simulink model "Single1"  (R2016a)
settings: Solver=FixedStepDiscrete  StartTime=0.0  StopTime=400e-9  FixedStep=SampleTime  RelTol=1e-3
values from neighbouring files (symbols this model uses):
  Rd = (3.6/4) * (0.95*0.82*(1 - (-0.0128*(Temp - 25))) * 18.2 / 295) + 1e-4    (= 0.11256119322)    [DPTThermalGaNModel.m]    (also in Thermal_CurrentVoltageGraph.m = (3.6/4) * (0.95*0.82*(1 - (-0.0128*(Temp(TempIndex) - 25))) )
  Rs = 3.6 * 0.238 * 0.82 * (1 - (-0.0128*(Temp - 25))) / 295 + 1e-4    (= 0.00629219525424)    [DPTThermalGaNModel.m]    (also in Thermal_CurrentVoltageGraph.m = 3.6 * 0.238 * 0.82 * (1 - (-0.0128*(Temp(TempIndex) - 25))) )
  Rss = 1e-3    (= 0.001)    [DPTThermalGaNModel.m]
  VpulseMax = 6    [DPTThermalGaNModel.m]
undefined symbols (not defined in the file or in its folder): Rgin
libraries: elec_lib x16, nesl_utility x15, fl_lib x14
settings Model: Creator=ugurm  LastModifiedBy=Furkan
settings OptimizationCC: EfficientMapNaN2IntZero=off
settings HardwareCC: TargetBitPerPointer=64  TargetLongLongMode=on  TargetIntDivRoundTo=Zero  TargetEndianess=LittleEndian  TargetWordSize=64  TargetHWDeviceType=MATLAB Host  ProdEqTarget=off
settings CodeAppCC: MaxIdLength=128
settings GRTTargetCC: GeneratePreprocessorConditionals=Use local settings  CombineOutputUpdateFcns=off  GRTInterface=on

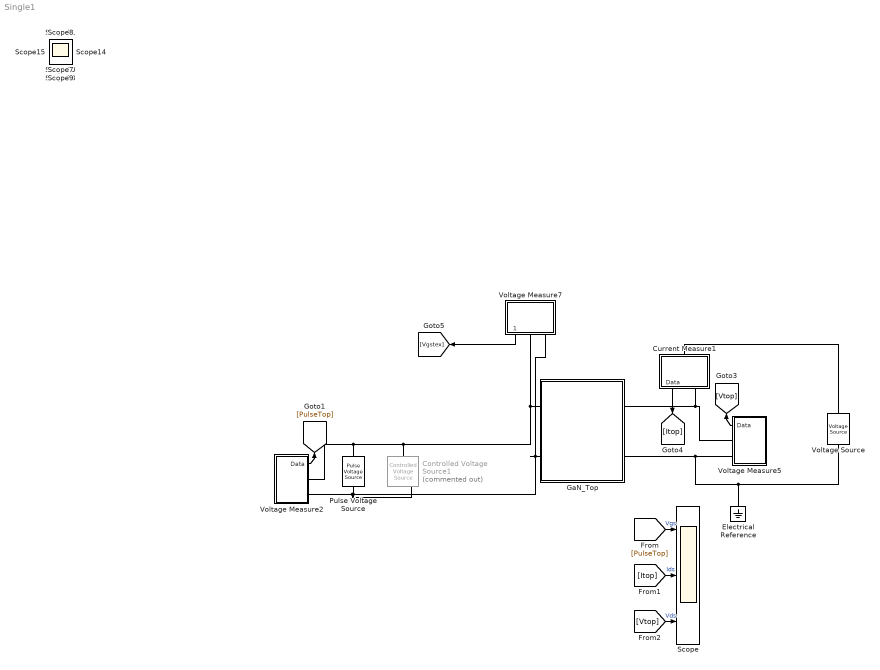
== system Single1 ==
  Controlled Voltage Source1 : fl_lib/Electrical/Electrical Sources/Controlled Voltage Source  Commented=on
  Current Measure1 : Subsystem
  Electrical Reference : fl_lib/Electrical/Electrical Elements/Electrical Reference
  GaN_Top : Subsystem
  Pulse Voltage Source : elec_lib/Additional Components/SPICE-Compatible Components/Sources/Pulse Voltage Source  V1=-3 V  V2=6 V  TD=50e-9 s  TR=1e-10 s  TF=1e-10 s  PW=150e-9 s  PER=500e-9 s
  Scope : Scope  NumInputPorts=3
  Voltage Measure2 : Subsystem
  Voltage Measure5 : Subsystem
  Voltage Measure7 : Subsystem
  Voltage Source : elec_lib/Sources/Voltage Source  dc_voltage=2 V  ac_voltage=0 V  ac_shift=0 deg  ac_frequency=60 Hz  noise_mode=0  PSD=0 V^2/Hz  sample_time=0.001 s  repeatability=1  auto_seed=3499211588  user_seed=0
  Scope{7..11,13..15} (8 alike) : Scope
  wires:
  Voltage Measure2/1(Data) -> [PulseTop]
  Voltage Measure5/1(Data) -> [Vtop]
  Current Measure1/1(Data) -> [Itop]
  Voltage Measure7/1(Data) -> [Vgstex]
  [PulseTop] -> Scope/1  "Vgs"
  [Itop] -> Scope/2  "Ids"
  [Vtop] -> Scope/3  "Vds"
  connections:
  GaN_Top/LConn1 -- Voltage Measure2/RConn1 -- Pulse Voltage Source/LConn1 -- Controlled Voltage Source1/LConn1 -- Voltage Measure7/RConn1
  GaN_Top/RConn1 -- Current Measure1/RConn1 -- Voltage Measure5/RConn1
  Pulse Voltage Source/RConn1 -- Controlled Voltage Source1/RConn2 -- Voltage Measure2/RConn2 -- GaN_Top/LConn2 -- Voltage Measure7/RConn2
  GaN_Top/RConn2 -- Electrical Reference/LConn1 -- Voltage Source/RConn1 -- Voltage Measure5/RConn2
  Voltage Source/LConn1 -- Current Measure1/LConn1

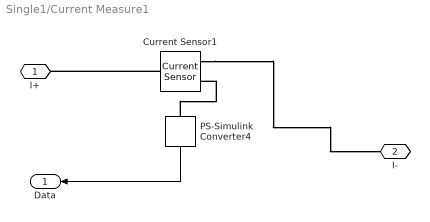
== system Single1/Current Measure1 ==
  Current Sensor1 : fl_lib/Electrical/Electrical Sensors/Current Sensor
  PS-Simulink Converter4 : nesl_utility/PS-Simulink Converter  PhysicalDomain=network_engine_domain  SubClassName=ps_output  LeftPortType=input  RightPortType=output  PseudoPeriodic=off  Frequencies=[]  Unit=1  AffineConversion=off
  I+ : PMIOPort  Port=1  Side=Left
  I- : PMIOPort  Port=2  Side=Right
  Data : Outport
  wires:
  PS-Simulink Converter4/1 -> Data/1
  connections:
  Current Sensor1/RConn2 -- I-/RConn1
  PS-Simulink Converter4/LConn1 -- Current Sensor1/RConn1
  Current Sensor1/LConn1 -- I+/RConn1

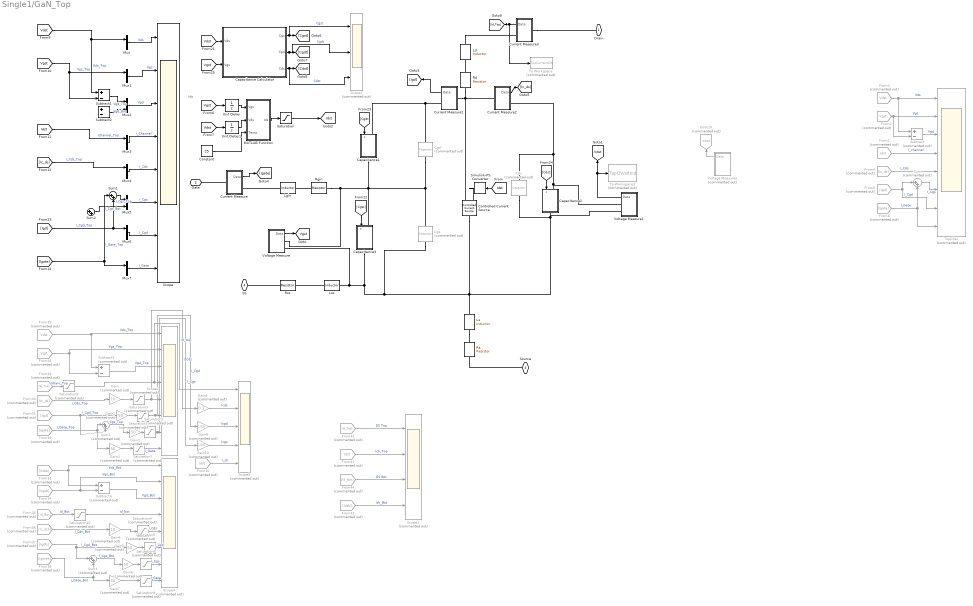
== system Single1/GaN_Top ==
  note: Ids
  Capacitance Calculator : Subsystem
  Capacitance1 : Subsystem
  Capacitance2 : Subsystem
  Capacitance3 : Subsystem
  Cds : elec_lib/Passive Devices/Capacitor  Commented=on  enable_table=0  c=Cds F  Cvec=[ 1e-5 1e-6 ] F  Vvec=[ 0 10 ] V  CV_table_symmetry=1  C_tol=5  enable_C_tol=0  tol_distribution=1  nSigma=4  r=1e-6 Ohm  g=0 1/Ohm  initV=VoltDSTop V  enable_operating_limits=0  operating_limit_action=2  max_working_voltage_range=[ -25 25 ] V  power_rating=1 W  enable_faults=0  fault_action=1  Cscale_faulted=100  R_faulted=0.001 Ohm  G_faulted=0 1/Ohm  tau_fault=0.001 s  enable_temporal_fault=0  t_fault=1 s  enable_behavioral_fault=0  max_permissible_voltage_range=[ -100 100 ] V  t_fail_on_voltage=1 s
  Cgd : elec_lib/Passive Devices/Capacitor  Commented=on  enable_table=0  c=Cgd F  Cvec=[ 1e-5 1e-6 ] F  Vvec=[ 0 10 ] V  CV_table_symmetry=1  C_tol=5  enable_C_tol=0  tol_distribution=1  nSigma=4  r=1e-6 Ohm  g=0 1/Ohm  initV=-VpulseMax V  enable_operating_limits=0  operating_limit_action=2  max_working_voltage_range=[ -25 25 ] V  power_rating=1 W  enable_faults=0  fault_action=1  Cscale_faulted=100  R_faulted=0.001 Ohm  G_faulted=0 1/Ohm  tau_fault=0.001 s  enable_temporal_fault=0  t_fault=1 s  enable_behavioral_fault=0  max_permissible_voltage_range=[ -100 100 ] V  t_fail_on_voltage=1 s
  Cgs : elec_lib/Passive Devices/Capacitor  Commented=on  enable_table=0  c=Cgs F  Cvec=[ 1e-5 1e-6 ] F  Vvec=[ 0 10 ] V  CV_table_symmetry=1  C_tol=5  enable_C_tol=0  tol_distribution=1  nSigma=4  r=1e-6 Ohm  g=0 1/Ohm  initV=VpulseMin V  enable_operating_limits=0  operating_limit_action=2  max_working_voltage_range=[ -25 25 ] V  power_rating=1 W  enable_faults=0  fault_action=1  Cscale_faulted=100  R_faulted=0.001 Ohm  G_faulted=0 1/Ohm  tau_fault=0.001 s  enable_temporal_fault=0  t_fault=1 s  enable_behavioral_fault=0  max_permissible_voltage_range=[ -100 100 ] V  t_fail_on_voltage=1 s
  Constant : Constant  Value=25
  Controlled Current Source : fl_lib/Electrical/Electrical Sources/Controlled Current Source
  Current Measure : Subsystem
  Current Measure1 : Subsystem
  Current Measure2 : Subsystem
  Current Measure3 : Subsystem
  From1 : From  Commented=on  GotoTag=Idst  TagVisibility=global
  From2 : From  Commented=on  GotoTag=Vgst  TagVisibility=global
  From28 : From  Commented=on  GotoTag=Vgst  TagVisibility=global
  From29 : From  Commented=on  GotoTag=Id_Top
  From3 : From  Commented=on  GotoTag=Vdst  TagVisibility=global
  From30 : From  Commented=on  GotoTag=Ic_ds
  From31 : From  Commented=on  GotoTag=Igd
  From32 : From  Commented=on  GotoTag=Igate
  From33 : From  Commented=on  GotoTag=Vdsb  TagVisibility=global
  From34 : From  Commented=on  GotoTag=Vgsb  TagVisibility=global
  From35 : From  Commented=on  GotoTag=Id_Bot  TagVisibility=global
  From36 : From  Commented=on  GotoTag=Ic_dsb  TagVisibility=global
  From37 : From  Commented=on  GotoTag=Igdb  TagVisibility=global
  From38 : From  Commented=on  GotoTag=Igateb  TagVisibility=global
  From39 : From  Commented=on  GotoTag=Vdst  TagVisibility=global
  From4 : From  Commented=on  GotoTag=Ic_ds
  From40 : From  Commented=on  GotoTag=Idst  TagVisibility=global
  From41 : From  Commented=on  GotoTag=Idst  TagVisibility=global
  From42 : From  Commented=on  GotoTag=Idsb  TagVisibility=global
  From43 : From  Commented=on  GotoTag=Id_Top
  From44 : From  Commented=on  GotoTag=Id_Bot  TagVisibility=global
  From5 : From  Commented=on  GotoTag=Igd
  From8 : From  Commented=on  GotoTag=Igate
  Gain : Gain  Commented=on  Gain=10
  Gain{1..3,5..7} (6 alike) : Gain  Commented=on  Gain=50
  Gain10 : Gain  Commented=on  Gain=1/50
  Gain4 : Gain  Commented=on  Gain=10
  Gain8 : Gain  Commented=on  Gain=0.1
  Gain9 : Gain  Commented=on  Gain=1/50
  Goto10 : Goto  Commented=on  GotoTag=Vdsit  TagVisibility=global
  Ld : elec_lib/Passive Devices/Inductor  l=Ld H  L_tol=20  enable_L_tol=0  tol_distribution=1  nSigma=4  r=0 Ohm  g=1e-9 1/Ohm  initI=CurrDSTop A  enable_operating_limits=0  operating_limit_action=2  max_working_current=1 A  power_rating=1 W  enable_faults=0  fault_action=1  lambdaPercent=50  k_faulted=0.9999 Ohm  turnsShort=0  openCct=0  groundShort=0  groundShortG=0 1/Ohm  tau_fault=0.001 s  enable_temporal_fault=0  t_fault=1 s  enable_behavioral_fault=0  max_permissible_voltage=100 V  n_fail_on_voltage=1  max_permissible_current=1 A  t_fail_on_current=1 s
  "Lgin " : elec_lib/Passive Devices/Inductor  l=Lgin H  L_tol=20  enable_L_tol=0  tol_distribution=1  nSigma=4  r=0 Ohm  g=1e-9 1/Ohm  initI=0 A  enable_operating_limits=0  operating_limit_action=2  max_working_current=1 A  power_rating=1 W  enable_faults=0  fault_action=1  lambdaPercent=50  k_faulted=0.9999 Ohm  turnsShort=0  openCct=0  groundShort=0  groundShortG=0 1/Ohm  tau_fault=0.001 s  enable_temporal_fault=0  t_fault=1 s  enable_behavioral_fault=0  max_permissible_voltage=100 V  n_fail_on_voltage=1  max_permissible_current=1 A  t_fail_on_current=1 s
  Ls : elec_lib/Passive Devices/Inductor  l=Ls H  L_tol=20  enable_L_tol=0  tol_distribution=1  nSigma=4  r=0 Ohm  g=1e-9 1/Ohm  initI=CurrDSTop A  enable_operating_limits=0  operating_limit_action=2  max_working_current=1 A  power_rating=1 W  enable_faults=0  fault_action=1  lambdaPercent=50  k_faulted=0.9999 Ohm  turnsShort=0  openCct=0  groundShort=0  groundShortG=0 1/Ohm  tau_fault=0.001 s  enable_temporal_fault=0  t_fault=1 s  enable_behavioral_fault=0  max_permissible_voltage=100 V  n_fail_on_voltage=1  max_permissible_current=1 A  t_fail_on_current=1 s
  Lss : elec_lib/Passive Devices/Inductor  l=Lss H  L_tol=20  enable_L_tol=0  tol_distribution=1  nSigma=4  r=0 Ohm  g=1e-9 1/Ohm  initI=0 A  enable_operating_limits=0  operating_limit_action=2  max_working_current=1 A  power_rating=1 W  enable_faults=0  fault_action=1  lambdaPercent=50  k_faulted=0.9999 Ohm  turnsShort=0  openCct=0  groundShort=0  groundShortG=0 1/Ohm  tau_fault=0.001 s  enable_temporal_fault=0  t_fault=1 s  enable_behavioral_fault=0  max_permissible_voltage=100 V  n_fail_on_voltage=1  max_permissible_current=1 A  t_fail_on_current=1 s
  MATLAB Function : MATLAB Function  TreatAsAtomicUnit=on
  Mux{,1..7} (8 alike) : Mux  Inputs=2
  Rd : elec_lib/Passive Devices/Resistor  R=Rd Ohm  R_tol=5  enable_R_tol=0  tol_distribution=1  nSigma=4  enable_operating_limits=0  operating_limit_action=2  max_working_voltage=100 V  power_rating=1 W  enable_faults=0  fault_action=1  R_faulted=Inf Ohm  enable_temporal_fault=0  t_fault=1 s  enable_behavioral_fault=0  max_permissible_current=1 A  t_fail_on_current=1 s  noise_mode=0  sample_time=0.001 s  repeatability=1  auto_seed=1426435484  user_seed=0  Tdevice=25 degC  alpha=0.00393 1/K  Tmeas=25 degC  thermal_mass=100 J/K  initial_temperature=25 degC  power_derating_T1=70 degC  power_derating_T2=155 degC  operating_temperature_range_vec=[ -50 150 ] degC
  "Rgin " : elec_lib/Passive Devices/Resistor  R=Rgin Ohm  R_tol=5  enable_R_tol=0  tol_distribution=1  nSigma=4  enable_operating_limits=0  operating_limit_action=2  max_working_voltage=100 V  power_rating=1 W  enable_faults=0  fault_action=1  R_faulted=Inf Ohm  enable_temporal_fault=0  t_fault=1 s  enable_behavioral_fault=0  max_permissible_current=1 A  t_fail_on_current=1 s  noise_mode=0  sample_time=0.001 s  repeatability=1  auto_seed=2715962282  user_seed=0  Tdevice=25 degC  alpha=0.00393 1/K  Tmeas=25 degC  thermal_mass=100 J/K  initial_temperature=25 degC  power_derating_T1=70 degC  power_derating_T2=155 degC  operating_temperature_range_vec=[ -50 150 ] degC
  Rs : elec_lib/Passive Devices/Resistor  R=Rs Ohm  R_tol=5  enable_R_tol=0  tol_distribution=1  nSigma=4  enable_operating_limits=0  operating_limit_action=2  max_working_voltage=100 V  power_rating=1 W  enable_faults=0  fault_action=1  R_faulted=Inf Ohm  enable_temporal_fault=0  t_fault=1 s  enable_behavioral_fault=0  max_permissible_current=1 A  t_fail_on_current=1 s  noise_mode=0  sample_time=0.001 s  repeatability=1  auto_seed=3428974147  user_seed=0  Tdevice=25 degC  alpha=0.00393 1/K  Tmeas=25 degC  thermal_mass=100 J/K  initial_temperature=25 degC  power_derating_T1=70 degC  power_derating_T2=155 degC  operating_temperature_range_vec=[ -50 150 ] degC
  Rss : elec_lib/Passive Devices/Resistor  R=Rss Ohm  R_tol=5  enable_R_tol=0  tol_distribution=1  nSigma=4  enable_operating_limits=0  operating_limit_action=2  max_working_voltage=100 V  power_rating=1 W  enable_faults=0  fault_action=1  R_faulted=Inf Ohm  enable_temporal_fault=0  t_fault=1 s  enable_behavioral_fault=0  max_permissible_current=1 A  t_fail_on_current=1 s  noise_mode=0  sample_time=0.001 s  repeatability=1  auto_seed=299565776  user_seed=0  Tdevice=25 degC  alpha=0.00393 1/K  Tmeas=25 degC  thermal_mass=100 J/K  initial_temperature=25 degC  power_derating_T1=70 degC  power_derating_T2=155 degC  operating_temperature_range_vec=[ -50 150 ] degC
  Saturation : Saturate  UpperLimit=200  LowerLimit=-200
  Saturation{1..2,5..10} (8 alike) : Saturate  Commented=on  UpperLimit=100  LowerLimit=-100
  Saturation3 : Saturate  Commented=on  UpperLimit=250  LowerLimit=-100
  Saturation4 : Saturate  Commented=on  UpperLimit=250  LowerLimit=-100
  Scope : Scope  NumInputPorts=8
  Scope1 : Scope  Commented=on  NumInputPorts=3
  Scope2 : Scope  Commented=on  NumInputPorts=8
  Scope3 : Scope  Commented=on  NumInputPorts=4
  Scope4 : Scope  Commented=on  NumInputPorts=8
  Scope5 : Scope  Commented=on  NumInputPorts=5
  Simulink-PS Converter : nesl_utility/Simulink-PS Converter  PhysicalDomain=network_engine_domain  SubClassName=ps_input  LeftPortType=input  RightPortType=output  PseudoPeriodic=off  Frequencies=[]  NoiseDistribution=none  NoiseParameters=[]  Unit=1  AffineConversion=off  InputFiltering=off  SimscapeFilterOrder=1  InputFilterTimeConstant=0.001  UdotUserProvided=1
  Subtract : Sum  Commented=on  Inputs=+-
  Subtract1 : Sum  Inputs=+-
  Subtract2 : Sum  Inputs=+-
  Subtract3 : Sum  Commented=on  Inputs=+-
  Subtract4 : Sum  Commented=on  Inputs=+-
  Sum : Sum  Commented=on  Inputs=|++
  Sum1 : Sum  Inputs=|++
  Sum2 : Sum  Inputs=|++
  Sum3 : Sum  Commented=on  Inputs=|++
  Sum4 : Sum  Commented=on  Inputs=|++
  To Workspace : ToWorkspace  Commented=on  VariableName=TopCurrentDS  SampleTime=-1
      settings: Save2DSignal=2-D array (concatenate along first dimension)
  To Workspace3 : ToWorkspace  Commented=on  VariableName=TopChVoltInd  SampleTime=-1
      settings: Save2DSignal=2-D array (concatenate along first dimension)
  TopChar : Scope  Commented=on  NumInputPorts=8
  Unit Delay : UnitDelay  SampleTime=-1
  Unit Delay1 : UnitDelay  SampleTime=-1
  Voltage Measure : Subsystem
  Voltage Measure1 : Subsystem
  Voltage Measure2 : Subsystem  Commented=on
  Drain : PMIOPort  Port=1  Side=Right
  Gate : PMIOPort  Port=2  Side=Left
  Source : PMIOPort  Port=3  Side=Right
  SS : PMIOPort  Port=4  Side=Left
  tag scope: Idst=global, Vdst=global, Vgst=global
  wires:
  [Vgst] -> Unit Delay/1
  MATLAB Function/1(Ids) -> Saturation/1
  Unit Delay/1 -> MATLAB Function/1(Vgs)
  [Idst] -> Simulink-PS Converter/1
  From2/1 -> Subtract/2, TopChar/2  "Vgs"
  From3/1 -> Subtract/1, TopChar/1  "Vds"
  From1/1 -> TopChar/4  "I_channel"
  Subtract/1 -> TopChar/3  "Vgd"
  Current Measure1/1(Data) -> [Igd]
  Current Measure2/1(Data) -> [Ic_ds]
  From5/1 -> TopChar/7, Sum/1  "I_Cgd"
  From8/1 -> TopChar/8, Sum/2  "I_Gate"
  From4/1 -> TopChar/5  "I_Cds"
  Sum/1 -> TopChar/6  "I_Cgs"
  Current Measure/1(Data) -> [Igate]
  Voltage Measure/1(Data) -> [Vgst]
  [Vdst] -> Mux/1, Subtract1/1  "Vds_Top"
  [Vgst] -> Mux1/1, Subtract1/2  "Vgs_Top"
  [Ic_ds] -> Mux4/1  "I_Cds_Top"
  [Igd] -> Mux6/1, Sum1/2  "I_Cgd_Top"
  [Igate] -> Mux7/1, Sum1/1  "I_Gate_Top"
  Sum1/1 -> Mux5/1  "I_Cgs_Top"
  ? -> Subtract2/1, Mux/2  "Vds_Bot"
  ? -> Mux1/2, Subtract2/2  "Vgs_Bot"
  ? -> Mux4/2  "I_Cds_Bot"
  ? -> Mux6/2, Sum2/1  "I_Cgd_Bot"
  ? -> Mux7/2, Sum2/2  "I_Gate_Bot"
  Sum2/1 -> Mux5/2  "I_Cgs_Bot"
  Subtract1/1 -> Mux2/1  "Vgd_Top"
  Subtract2/1 -> Mux2/2  "Vgd_Bot"
  [Idst] -> Mux3/1  "Ichannel_Top"
  ? -> Mux3/2  "Ichannel_Bot"
  Mux7/1 -> Scope/8  "I_Gate"
  Mux6/1 -> Scope/7  "I_Cgd"
  Mux5/1 -> Scope/6  "I_Cgs"
  Mux4/1 -> Scope/5  "I_Cds"
  Mux3/1 -> Scope/4  "I_Channel"
  Mux2/1 -> Scope/3  "Vgd"
  Mux1/1 -> Scope/2  "Vgs"
  Mux/1 -> Scope/1  "Vds"
  [Vdst] -> Capacitance Calculator/1(Vds)
  Capacitance Calculator/1(Cgs) -> Scope1/1, [Cgst]  "Cgst"
  Capacitance Calculator/2(Cgd) -> Scope1/2, [Cgdt]  "Cgdt"
  Capacitance Calculator/3(Cds) -> Scope1/3, [Cdst]  "Cdst"
  [Cgst] -> Capacitance3/1(c)
  [Cgdt] -> Capacitance1/1(c)
  [Cdst] -> Capacitance2/1(c)
  From39/1 -> Scope2/1, Subtract3/1  "Vds_Top"
  From28/1 -> Scope2/2, Subtract3/2  "Vgs_Top"
  From30/1 -> Gain/1  "I_Cds_Top"
  From31/1 -> Sum3/2, Gain1/1  "I_Cgd_Top"
  From32/1 -> Gain3/1, Sum3/1  "I_Gate_Top"
  From33/1 -> Scope4/1, Subtract4/1  "Vds_Bot"
  From34/1 -> Scope4/2, Subtract4/2  "Vgs_Bot"
  From36/1 -> Gain4/1  "I_Cds_Bot"
  From37/1 -> Sum4/1, Gain5/1  "I_Cgd_Bot"
  From38/1 -> Gain7/1, Sum4/2  "I_Gate_Bot"
  Subtract3/1 -> Scope2/3  "Vgd_Top"
  Subtract4/1 -> Scope4/3  "Vgd_Bot"
  From29/1 -> Saturation9/1  "Idrain_Top"
  From35/1 -> Saturation10/1  "Id_Bot"
  Sum4/1 -> Gain6/1  "I_Cgs_Bot"
  Gain/1 -> Saturation3/1
  Gain1/1 -> Saturation2/1
  Sum3/1 -> Gain2/1  "I_Cgs_Top"
  Gain3/1 -> Saturation7/1
  Gain4/1 -> Saturation4/1
  Gain6/1 -> Saturation6/1
  Gain7/1 -> Saturation8/1
  Gain2/1 -> Saturation1/1
  Saturation1/1 -> Gain10/1, Scope2/7  "I_Cgs"
  Saturation2/1 -> Gain9/1, Scope2/6  "I_Cgd"
  Saturation3/1 -> Gain8/1, Scope2/5  "I_Cds"
  Saturation4/1 -> Scope4/5  "I_Cds"
  Saturation5/1 -> Scope4/6  "I_Cgd"
  Gain5/1 -> Saturation5/1
  Saturation6/1 -> Scope4/7  "I_Cgs"
  Saturation7/1 -> Scope2/8  "I_Gate"
  Saturation8/1 -> Scope4/8  "I_Gate"
  Current Measure3/1(Data) -> To Workspace/1, [Id_Top]
  Saturation9/1 -> Scope5/1, Scope2/4  "Id_top"
  Saturation10/1 -> Scope4/4  "Id_bot"
  Gain8/1 -> Scope5/2  "Icds"
  Gain9/1 -> Scope5/3  "Icgd"
  Gain10/1 -> Scope5/4  "Icgs"
  From40/1 -> Scope5/5  "I_ch"
  From41/1 -> Scope3/2  "Ich_Top"
  From42/1 -> Scope3/4  "Ich_Bot"
  [Vdst] -> Unit Delay1/1
  Unit Delay1/1 -> MATLAB Function/2(Vds)
  Voltage Measure2/1(Data) -> Goto10/1
  Saturation/1 -> [Idst]
  Voltage Measure1/1(Data) -> To Workspace3/1, [Vdst]
  From43/1 -> Scope3/1  "DS Top"
  From44/1 -> Scope3/3  "DS Bot"
  [Vgst] -> Capacitance Calculator/2(Vgs)
  Constant/1 -> MATLAB Function/3(Temp)
  connections:
  Capacitance1/RConn1 -- Voltage Measure/RConn1 -- "Rgin "/LConn1 -- Cgs/LConn1 -- Cgd/RConn1 -- Capacitance3/LConn1
  Simulink-PS Converter/RConn1 -- Controlled Current Source/RConn1
  Current Measure/LConn1 -- Gate/RConn1
  Capacitance1/LConn1 -- Current Measure1/RConn1 -- Cgd/LConn1
  Capacitance2/LConn1 -- Voltage Measure1/RConn1 -- Cds/LConn1 -- Current Measure2/RConn1
  Current Measure3/LConn1 -- Drain/RConn1
  "Lgin "/LConn1 -- Current Measure/RConn1
  Rss/LConn1 -- SS/RConn1
  Capacitance3/RConn1 -- Controlled Current Source/LConn1 -- Ls/LConn1 -- Cds/RConn1 -- Voltage Measure1/RConn2 -- Capacitance2/RConn1 -- Cgs/RConn1 -- Voltage Measure/RConn2 -- Lss/RConn1
  Source/RConn1 -- Rs/RConn1
  Rd/LConn1 -- Ld/RConn1
  Lss/LConn1 -- Rss/RConn1
  Ls/RConn1 -- Rs/LConn1
  Current Measure3/RConn1 -- Ld/LConn1
  "Rgin "/RConn1 -- "Lgin "/RConn1
  Current Measure2/LConn1 -- Controlled Current Source/RConn2 -- Rd/RConn1 -- Current Measure1/LConn1

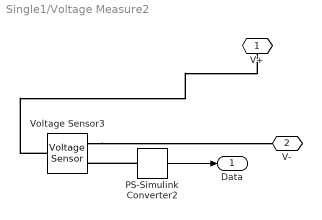
== system Single1/Voltage Measure2 ==
  PS-Simulink Converter2 : nesl_utility/PS-Simulink Converter  PhysicalDomain=network_engine_domain  SubClassName=ps_output  LeftPortType=input  RightPortType=output  PseudoPeriodic=off  Frequencies=[]  Unit=1  AffineConversion=off
  Voltage Sensor3 : fl_lib/Electrical/Electrical Sensors/Voltage Sensor
  V+ : PMIOPort  Port=1  Side=Right
  V- : PMIOPort  Port=2  Side=Right
  Data : Outport
  wires:
  PS-Simulink Converter2/1 -> Data/1
  connections:
  Voltage Sensor3/LConn1 -- V+/RConn1
  Voltage Sensor3/RConn2 -- V-/RConn1
  PS-Simulink Converter2/LConn1 -- Voltage Sensor3/RConn1

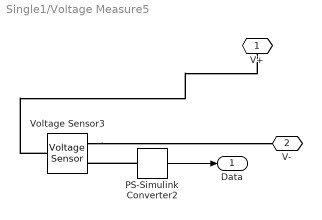
== system Single1/Voltage Measure5 ==
  PS-Simulink Converter2 : nesl_utility/PS-Simulink Converter  PhysicalDomain=network_engine_domain  SubClassName=ps_output  LeftPortType=input  RightPortType=output  PseudoPeriodic=off  Frequencies=[]  Unit=1  AffineConversion=off
  Voltage Sensor3 : fl_lib/Electrical/Electrical Sensors/Voltage Sensor
  V+ : PMIOPort  Port=1  Side=Right
  V- : PMIOPort  Port=2  Side=Right
  Data : Outport
  wires:
  PS-Simulink Converter2/1 -> Data/1
  connections:
  PS-Simulink Converter2/LConn1 -- Voltage Sensor3/RConn1
  Voltage Sensor3/RConn2 -- V-/RConn1
  Voltage Sensor3/LConn1 -- V+/RConn1

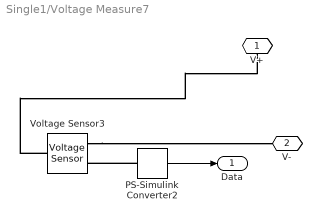
== system Single1/Voltage Measure7 ==
  PS-Simulink Converter2 : nesl_utility/PS-Simulink Converter  PhysicalDomain=network_engine_domain  SubClassName=ps_output  LeftPortType=input  RightPortType=output  PseudoPeriodic=off  Frequencies=[]  Unit=1  AffineConversion=off
  Voltage Sensor3 : fl_lib/Electrical/Electrical Sensors/Voltage Sensor
  V+ : PMIOPort  Port=1  Side=Right
  V- : PMIOPort  Port=2  Side=Right
  Data : Outport
  wires:
  PS-Simulink Converter2/1 -> Data/1
  connections:
  PS-Simulink Converter2/LConn1 -- Voltage Sensor3/RConn1
  Voltage Sensor3/RConn2 -- V-/RConn1
  Voltage Sensor3/LConn1 -- V+/RConn1

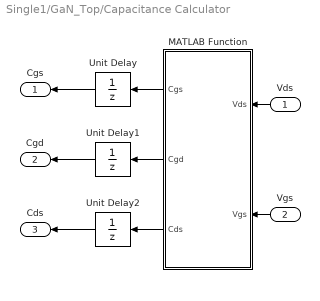
== system Single1/GaN_Top/Capacitance Calculator ==
  Vds : Inport
  Vgs : Inport  Port=2
  MATLAB Function : MATLAB Function  TreatAsAtomicUnit=on
  Unit Delay : UnitDelay  InitialCondition=258e-12  SampleTime=-1
  Unit Delay1 : UnitDelay  InitialCondition=63e-12  SampleTime=-1
  Unit Delay2 : UnitDelay  InitialCondition=2e-12  SampleTime=-1
  Cgs : Outport
  Cgd : Outport  Port=2
  Cds : Outport  Port=3
  wires:
  Vds/1 -> MATLAB Function/1(Vds)
  MATLAB Function/1(Cgs) -> Unit Delay/1
  MATLAB Function/2(Cgd) -> Unit Delay1/1
  MATLAB Function/3(Cds) -> Unit Delay2/1
  Unit Delay/1 -> Cgs/1
  Unit Delay1/1 -> Cgd/1
  Unit Delay2/1 -> Cds/1
  Vgs/1 -> MATLAB Function/2(Vgs)

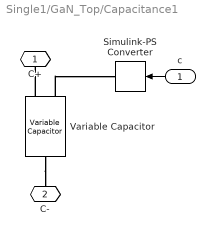
== system Single1/GaN_Top/Capacitance1 ==
  c : Inport
  Simulink-PS Converter : nesl_utility/Simulink-PS Converter  PhysicalDomain=network_engine_domain  SubClassName=ps_input  LeftPortType=input  RightPortType=output  PseudoPeriodic=off  Frequencies=[]  NoiseDistribution=none  NoiseParameters=[]  Unit=1  AffineConversion=off  InputFiltering=off  SimscapeFilterOrder=1  InputFilterTimeConstant=0.001  UdotUserProvided=1
  Variable Capacitor : elec_lib/Passive Devices/Variable Capacitor  prm=2  Cmin=1e-13 F  r=1e-6 Ohm  v0=VoltGDTop V  q0=0 c
  C+ : PMIOPort  Port=1  Side=Left
  C- : PMIOPort  Port=2  Side=Right
  wires:
  c/1 -> Simulink-PS Converter/1
  connections:
  Variable Capacitor/LConn1 -- Simulink-PS Converter/RConn1
  Variable Capacitor/LConn2 -- C+/RConn1
  Variable Capacitor/RConn1 -- C-/RConn1

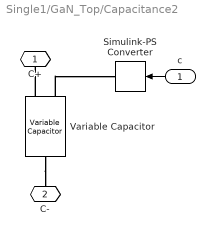
== system Single1/GaN_Top/Capacitance2 ==
  c : Inport
  Simulink-PS Converter : nesl_utility/Simulink-PS Converter  PhysicalDomain=network_engine_domain  SubClassName=ps_input  LeftPortType=input  RightPortType=output  PseudoPeriodic=off  Frequencies=[]  NoiseDistribution=none  NoiseParameters=[]  Unit=1  AffineConversion=off  InputFiltering=off  SimscapeFilterOrder=1  InputFilterTimeConstant=0.001  UdotUserProvided=1
  Variable Capacitor : elec_lib/Passive Devices/Variable Capacitor  prm=2  Cmin=1e-13 F  r=1e-6 Ohm  v0=VoltDSTop V  q0=0 c
  C+ : PMIOPort  Port=1  Side=Left
  C- : PMIOPort  Port=2  Side=Right
  wires:
  c/1 -> Simulink-PS Converter/1
  connections:
  Variable Capacitor/RConn1 -- C-/RConn1
  Variable Capacitor/LConn2 -- C+/RConn1
  Variable Capacitor/LConn1 -- Simulink-PS Converter/RConn1

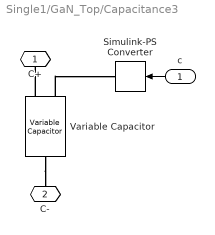
== system Single1/GaN_Top/Capacitance3 ==
  c : Inport
  Simulink-PS Converter : nesl_utility/Simulink-PS Converter  PhysicalDomain=network_engine_domain  SubClassName=ps_input  LeftPortType=input  RightPortType=output  PseudoPeriodic=off  Frequencies=[]  NoiseDistribution=none  NoiseParameters=[]  Unit=1  AffineConversion=off  InputFiltering=off  SimscapeFilterOrder=1  InputFilterTimeConstant=0.001  UdotUserProvided=1
  Variable Capacitor : elec_lib/Passive Devices/Variable Capacitor  prm=2  Cmin=1e-13 F  r=1e-6 Ohm  v0=VoltGSTop V  q0=0 c
  C+ : PMIOPort  Port=1  Side=Left
  C- : PMIOPort  Port=2  Side=Right
  wires:
  c/1 -> Simulink-PS Converter/1
  connections:
  Variable Capacitor/RConn1 -- C-/RConn1
  Variable Capacitor/LConn2 -- C+/RConn1
  Variable Capacitor/LConn1 -- Simulink-PS Converter/RConn1

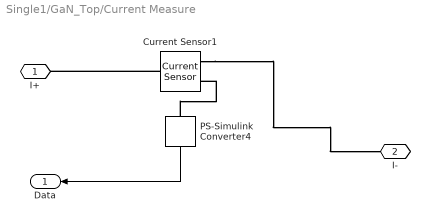
== system Single1/GaN_Top/Current Measure ==
  Current Sensor1 : fl_lib/Electrical/Electrical Sensors/Current Sensor
  PS-Simulink Converter4 : nesl_utility/PS-Simulink Converter  PhysicalDomain=network_engine_domain  SubClassName=ps_output  LeftPortType=input  RightPortType=output  PseudoPeriodic=off  Frequencies=[]  Unit=1  AffineConversion=off
  I+ : PMIOPort  Port=1  Side=Left
  I- : PMIOPort  Port=2  Side=Right
  Data : Outport
  wires:
  PS-Simulink Converter4/1 -> Data/1
  connections:
  Current Sensor1/RConn2 -- I-/RConn1
  PS-Simulink Converter4/LConn1 -- Current Sensor1/RConn1
  Current Sensor1/LConn1 -- I+/RConn1

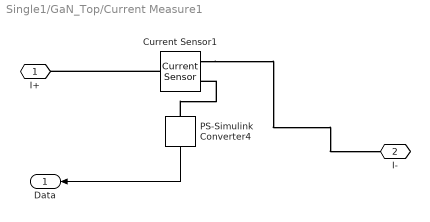
== system Single1/GaN_Top/Current Measure1 ==
  Current Sensor1 : fl_lib/Electrical/Electrical Sensors/Current Sensor
  PS-Simulink Converter4 : nesl_utility/PS-Simulink Converter  PhysicalDomain=network_engine_domain  SubClassName=ps_output  LeftPortType=input  RightPortType=output  PseudoPeriodic=off  Frequencies=[]  Unit=1  AffineConversion=off
  I+ : PMIOPort  Port=1  Side=Left
  I- : PMIOPort  Port=2  Side=Right
  Data : Outport
  wires:
  PS-Simulink Converter4/1 -> Data/1
  connections:
  Current Sensor1/LConn1 -- I+/RConn1
  PS-Simulink Converter4/LConn1 -- Current Sensor1/RConn1
  Current Sensor1/RConn2 -- I-/RConn1

== system Single1/GaN_Top/Current Measure2 ==
  Current Sensor1 : fl_lib/Electrical/Electrical Sensors/Current Sensor
  PS-Simulink Converter4 : nesl_utility/PS-Simulink Converter  PhysicalDomain=network_engine_domain  SubClassName=ps_output  LeftPortType=input  RightPortType=output  PseudoPeriodic=off  Frequencies=[]  Unit=1  AffineConversion=off
  I+ : PMIOPort  Port=1  Side=Left
  I- : PMIOPort  Port=2  Side=Right
  Data : Outport
  wires:
  PS-Simulink Converter4/1 -> Data/1
  connections:
  Current Sensor1/RConn2 -- I-/RConn1
  PS-Simulink Converter4/LConn1 -- Current Sensor1/RConn1
  Current Sensor1/LConn1 -- I+/RConn1

== system Single1/GaN_Top/Current Measure3 ==
  Current Sensor1 : fl_lib/Electrical/Electrical Sensors/Current Sensor
  PS-Simulink Converter4 : nesl_utility/PS-Simulink Converter  PhysicalDomain=network_engine_domain  SubClassName=ps_output  LeftPortType=input  RightPortType=output  PseudoPeriodic=off  Frequencies=[]  Unit=1  AffineConversion=off
  I+ : PMIOPort  Port=1  Side=Left
  I- : PMIOPort  Port=2  Side=Right
  Data : Outport
  wires:
  PS-Simulink Converter4/1 -> Data/1
  connections:
  Current Sensor1/RConn2 -- I-/RConn1
  PS-Simulink Converter4/LConn1 -- Current Sensor1/RConn1
  Current Sensor1/LConn1 -- I+/RConn1

== system Single1/GaN_Top/Voltage Measure ==
  PS-Simulink Converter2 : nesl_utility/PS-Simulink Converter  PhysicalDomain=network_engine_domain  SubClassName=ps_output  LeftPortType=input  RightPortType=output  PseudoPeriodic=off  Frequencies=[]  Unit=1  AffineConversion=off
  Voltage Sensor3 : fl_lib/Electrical/Electrical Sensors/Voltage Sensor
  V+ : PMIOPort  Port=1  Side=Right
  V- : PMIOPort  Port=2  Side=Right
  Data : Outport
  wires:
  PS-Simulink Converter2/1 -> Data/1
  connections:
  PS-Simulink Converter2/LConn1 -- Voltage Sensor3/RConn1
  Voltage Sensor3/RConn2 -- V-/RConn1
  Voltage Sensor3/LConn1 -- V+/RConn1

== system Single1/GaN_Top/Voltage Measure1 ==
  PS-Simulink Converter2 : nesl_utility/PS-Simulink Converter  PhysicalDomain=network_engine_domain  SubClassName=ps_output  LeftPortType=input  RightPortType=output  PseudoPeriodic=off  Frequencies=[]  Unit=1  AffineConversion=off
  Voltage Sensor3 : fl_lib/Electrical/Electrical Sensors/Voltage Sensor
  V+ : PMIOPort  Port=1  Side=Right
  V- : PMIOPort  Port=2  Side=Right
  Data : Outport
  wires:
  PS-Simulink Converter2/1 -> Data/1
  connections:
  Voltage Sensor3/LConn1 -- V+/RConn1
  Voltage Sensor3/RConn2 -- V-/RConn1
  PS-Simulink Converter2/LConn1 -- Voltage Sensor3/RConn1

== system Single1/GaN_Top/Voltage Measure2 ==
  PS-Simulink Converter2 : nesl_utility/PS-Simulink Converter  PhysicalDomain=network_engine_domain  SubClassName=ps_output  LeftPortType=input  RightPortType=output  PseudoPeriodic=off  Frequencies=[]  Unit=1  AffineConversion=off
  Voltage Sensor3 : fl_lib/Electrical/Electrical Sensors/Voltage Sensor
  V+ : PMIOPort  Port=1  Side=Right
  V- : PMIOPort  Port=2  Side=Right
  Data : Outport
  wires:
  PS-Simulink Converter2/1 -> Data/1
  connections:
  PS-Simulink Converter2/LConn1 -- Voltage Sensor3/RConn1
  Voltage Sensor3/RConn2 -- V-/RConn1
  Voltage Sensor3/LConn1 -- V+/RConn1

== matlab function Single1/GaN_Top/MATLAB Function ==
  data: Vgs input; Ids output; Vds input; Temp input
function Ids = fcn(Vgs,Vds,Temp)
%#codegen
% K1 = 0.283;
% b1 = 2.035;
% c1 = 0.124;
% d1 = 1.159;
% e1 = -0.204;
% m1 = 30.972;
% n1 = -4.48;
% K2 = 7.114;
% b2 = 2.054;
% c2 = 0.153;
% Vgs = 6;
% Vds = -0.045;
Vgd = Vgs - Vds;
cur = 4.5056641;
K = cur * 0.8 * ((Temp - 25 + 273)/300)^(-2.7);
x0 = 0.31 ;
x1 = 0.255;
slp = 2;


% if Vds>0
%     Ids = K1*log(1+exp((Vgs-b1)/c1))*((m1+n1*Vgs)*Vds)/(1+(d1+e1*Vgs)*Vds);
% else
% 
%     Ids = -K2*log(1+exp((Vgd-b2)/c2))*(-Vds/(1-Vds));
% end
if Vds>0
    Ids = K*log(1+exp(26*(Vgs-1.7)/slp))*(Vds)/((1+max((x0+x1*(Vgs+4.1)),0.2)*(Vds)));
else

    Ids = -K*log(1+exp(26*(Vgd-1.7)/slp))*(-Vds)/(1+max((x0+x1*(Vgd+6.1)),0.2)*(-Vds));
end

== matlab function Single1/GaN_Top/Capacitance Calculator/MATLAB Function ==
  data: Vds input; Cgs output; Cgd output; Cds output; Vgs input
function [Cgs,Cgd,Cds]= fcn(Vds,Vgs)
%#codegen
% Vdc = 400;
% VpulseMax = 6;
% VpulseMin = -3;
% Vdsgs = (Vdc/(VpulseMax - VpulseMin))*(Vgs + VpulseMin);
Vds = abs(Vds);
%% Crss calculation
       a1 =   2.519e+14;
       b1 =      -345.7;
       c1 =       63.76;
       a2 =       27.99;
       b2 =       12.86;
       c2 =       18.29;
       a3 =       8.666;
       b3 =       33.93;
       c3 =       9.161;
       a4 =       1.502;
       b4 =       125.5;
       c4 =       121.9;
       a5 =      0.6563;
       b5 =         500;
       c5 =       34.57;
       a6 =        1.98;
       b6 =       408.2;
       c6 =       134.7;
Crss = a1.*exp(-((Vds-b1)./c1).^2) + a2.*exp(-((Vds-b2)./c2).^2) + a3*exp(-((Vds-b3)./c3).^2)...
   + a4.*exp(-((Vds-b4)./c4).^2) +a5.*exp(-((Vds-b5)./c5).^2) +a6.*exp(-((Vds-b6)./c6).^2);
Crss = Crss*1e-12;
%% Ciss Calculation
%        a1 =        1167;
%        b1 =      -115.8;
%        c1 =       60.96;
%        a2 =       269.7;
%        b2 =       -5402;
%        c2 =   4.243e+04;
%        a3 =        3.61;
%        b3 =       238.5;
%        c3 =       2.507;
%        a4 =       1.036;
%        b4 =       175.8;
%        c4 =       16.81;
%        a5 =       1.571;
%        b5 =         263;
%        c5 =       3.586;
%        a6 =      -1.174;
%        b6 =       238.2;
%        c6 =       25.85;
       a1 =        267.6;
       b1 =      2.007;
       c1 =       0.4734;
       a2 =       240.1;
       b2 =       3.049;
       c2 =      1.104;
       a3 =        -1336;
       b3 =       7.803;
       c3 =       9.331;
       a4 =       -250.6;
       b4 =       7.082;
       c4 =       1.715;
       a5 =       -2352;
       b5 =         11.25;
       c5 =       3.184;
       a6 =      8.572e13;
       b6 =       340.6;
       c6 =       67.72;
Ciss = a1.*exp(-((Vgs-b1)./c1).^2) + a2.*exp(-((Vgs-b2)./c2).^2) + a3*exp(-((Vgs-b3)./c3).^2)...
   + a4.*exp(-((Vgs-b4)./c4).^2) +a5.*exp(-((Vgs-b5)./c5).^2) +a6.*exp(-((Vgs-b6)./c6).^2);
Ciss = Ciss*1e-12;
%% Coss Calculation
       a1 =         328;
       b1 =       -8.43;
       c1 =       30.26;
       a2 =       115.8;
       b2 =        42.2;
       c2 =       7.341;
       a3 =       45.83;
       b3 =       59.01;
       c3 =       6.099;
       a4 =       183.1;
       b4 =        28.6;
       c4 =       16.39;
       a5 =       69.29;
       b5 =       154.4;
       c5 =        1511;
       a6 =       125.6;
       b6 =       22.68;
       c6 =       119.6;
Coss = a1.*exp(-((Vds-b1)./c1).^2) + a2.*exp(-((Vds-b2)./c2).^2) + a3*exp(-((Vds-b3)./c3).^2)...
   + a4.*exp(-((Vds-b4)./c4).^2) +a5.*exp(-((Vds-b5)./c5).^2) +a6.*exp(-((Vds-b6)./c6).^2);
Coss = Coss*1e-12;
%% Outputs
Cgs = Ciss - Crss;
Cds = Coss - Crss;
Cgd = Crss;
